simulink model "daolibai"  (Simulink 8.0)
settings: Solver=ode45  StartTime=0.0  StopTime=100  MinStep=1e-5  RelTol=1e-2
libraries: fuzblock x2
settings Model: Creator=fangzhen  LastModifiedBy=fangzhen
settings SolverCC: ZeroCrossControl=DisableAll
settings DataIOCC: SignalLoggingSaveFormat=ModelDataLogs
settings DebuggingCC: FcnCallInpInsideContextMsg=EnableAllAsWarning

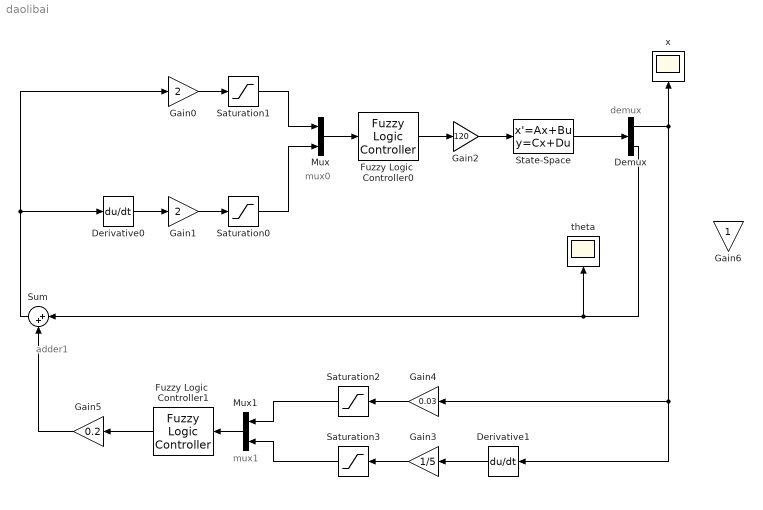
== system daolibai ==
  note: mux0
  note: mux1
  note: adder1
  note: demux
  Demux : Demux  Outputs=2
  Derivative0 : Derivative
  Derivative1 : Derivative
  Fuzzy Logic  Controller0 : fuzblock/Fuzzy Logic  Controller  fis=daolibait
  Fuzzy Logic  Controller1 : fuzblock/Fuzzy Logic  Controller  fis=daolibaix
  Gain0 : Gain  Gain=2
  Gain1 : Gain  Gain=2
  Gain2 : Gain  Gain=120
  Gain3 : Gain  Gain=1/5
  Gain4 : Gain  Gain=0.03
  Gain5 : Gain  Gain=0.2
  Gain6 : Gain
  Mux : Mux  Inputs=2
  Mux1 : Mux  Inputs=2
  Saturation{0..3} (4 alike) : Saturate  UpperLimit=2  LowerLimit=-2
  State-Space : StateSpace  A=[0,1,0,0; 0,0,10/12,0;0,0,0,1;0,0,100/12,0]  B=[0;1/9;0;1/12]  C=[1,0,0,0;0,0,1,0]  D=[0;0]  X0=[20;-4;-0.1;-0.10]  ContinuousStateAttributes='rad'
  Sum : Sum  Inputs=|++
  theta : Scope
      settings: TimeRange=200  YMin=-15  YMax=20
  x : Scope
      settings: TimeRange=200  YMin=-15  YMax=20
  wires:
  Derivative0/1 -> Gain1/1
  Gain0/1 -> Saturation1/1
  Gain1/1 -> Saturation0/1
  Mux/1 -> Fuzzy Logic  Controller0/1
  Fuzzy Logic  Controller0/1 -> Gain2/1
  Gain2/1 -> State-Space/1
  Saturation0/1 -> Mux/2
  Saturation1/1 -> Mux/1
  Derivative1/1 -> Gain3/1
  State-Space/1 -> Demux/1
  Gain4/1 -> Saturation2/1
  Gain3/1 -> Saturation3/1
  Mux1/1 -> Fuzzy Logic  Controller1/1
  Sum/1 -> Derivative0/1, Gain0/1
  Fuzzy Logic  Controller1/1 -> Gain5/1
  Gain5/1 -> Sum/2
  Saturation2/1 -> Mux1/1
  Saturation3/1 -> Mux1/2
  Demux/1 -> Derivative1/1, Gain4/1, x/1
  Demux/2 -> theta/1, Sum/1
